simulink library "WECSim_Lib"  (R2019b)
settings: Solver=ode45  StartTime=0.0  StopTime=10.0  RelTol=1e-3  EnableMultiTasking=on
undefined symbols (not defined in the file): body, constraint, mooring, pto, simu, waves, X, Y, Z
libraries: nesl_utility x168, sm_lib x94, vrlib x12
(part 5 of 6)

== system WECSim_Lib/Body Elements/Rigid Body/Hydrodynamic Body/Structure/Motion Sensor ==
  note: Measures the position, velocity, and acceleration of the follower (F) frame relative to the base (B) frame.
      | Ouputs a bus of 3 signals, each signal is a vector length 6.
  Angle : MATLAB Function  TreatAsAtomicUnit=on
  Bus Creator : BusCreator  Inputs=3
  Mux : Mux
  Mux1 : Mux  Inputs=6
  Mux2 : Mux  Inputs=6
  PS-Simulink Converter{,1..15} (16 alike) : nesl_utility/PS-Simulink Converter  PhysicalDomain=network_engine_domain  SubClassName=ps_output  LeftPortType=input  RightPortType=output  PseudoPeriodic=off  Frequencies=[]  Unit=1  AffineConversion=off
  Transform Sensor : sm_lib/Frames and Transforms/Transform Sensor  MeasurementFrame=World  SenseAngle=off  SenseAxis=off  SenseAngle1=off  SenseAngle2=off  SenseAngle3=off  SenseQ=on  SenseR=off  SenseOmegaX=on  SenseOmegaY=on  SenseOmegaZ=on  SenseOmega1=off  SenseOmega2=off  SenseOmega3=off  SenseQDot=off  SenseRDot=off  SenseAlphaX=on  SenseAlphaY=on  SenseAlphaZ=on  SenseAlpha1=off  SenseAlpha2=off  SenseAlpha3=off  SenseQDDot=off  SenseRDDot=off  SenseX=on  SenseY=on  SenseZ=on  SenseRad=off  SenseAzim=off  SenseDist=off  SenseInc=off  SenseXDot=on  SenseYDot=on  SenseZDot=on  SenseRadDot=off  SenseAzimDot=off  SenseDistDot=off  SenseIncDot=off  SenseXDDot=on  SenseYDDot=on  SenseZDDot=on  SenseRadDDot=off  SenseAzimDDot=off  SenseDistDDot=off  SenseIncDDot=off  BlockFunction=simmechanics.library.frames_transforms.transform_sensor
  F : PMIOPort  Side=Right
  B : PMIOPort  Port=2  Side=Left
  Response : Outport
  wires:
  Bus Creator/1 -> Response/1
  PS-Simulink Converter15/1 -> Mux2/3  "az"
  PS-Simulink Converter3/1 -> Mux1/6  "omegaz"
  PS-Simulink Converter11/1 -> Mux1/2  "vy"
  PS-Simulink Converter2/1 -> Mux1/5  "omegay"
  PS-Simulink Converter1/1 -> Mux1/4  "omegax"
  PS-Simulink Converter6/1 -> Mux2/6  "alphaz"
  PS-Simulink Converter5/1 -> Mux2/5  "alphay"
  PS-Simulink Converter9/1 -> Mux/3  "z"
  PS-Simulink Converter8/1 -> Mux/2  "y"
  PS-Simulink Converter7/1 -> Mux/1  "x"
  Angle/1(E) -> Mux/4
  Mux2/1 -> Bus Creator/3  "acc"
  Mux1/1 -> Bus Creator/2  "vel"
  Mux/1 -> Bus Creator/1  "disp"
  PS-Simulink Converter14/1 -> Mux2/2  "ay"
  PS-Simulink Converter13/1 -> Mux2/1  "ax"
  PS-Simulink Converter12/1 -> Mux1/3  "vz"
  PS-Simulink Converter10/1 -> Mux1/1  "vx"
  PS-Simulink Converter4/1 -> Mux2/4  "alphax"
  PS-Simulink Converter/1 -> Angle/1(Q)
  connections:
  PS-Simulink Converter3/LConn1 -- Transform Sensor/RConn5
  PS-Simulink Converter2/LConn1 -- Transform Sensor/RConn4
  PS-Simulink Converter1/LConn1 -- Transform Sensor/RConn3
  PS-Simulink Converter6/LConn1 -- Transform Sensor/RConn8
  PS-Simulink Converter5/LConn1 -- Transform Sensor/RConn7
  PS-Simulink Converter4/LConn1 -- Transform Sensor/RConn6
  PS-Simulink Converter7/LConn1 -- Transform Sensor/RConn9
  PS-Simulink Converter8/LConn1 -- Transform Sensor/RConn10
  PS-Simulink Converter9/LConn1 -- Transform Sensor/RConn11
  PS-Simulink Converter10/LConn1 -- Transform Sensor/RConn12
  PS-Simulink Converter11/LConn1 -- Transform Sensor/RConn13
  PS-Simulink Converter12/LConn1 -- Transform Sensor/RConn14
  PS-Simulink Converter13/LConn1 -- Transform Sensor/RConn15
  PS-Simulink Converter14/LConn1 -- Transform Sensor/RConn16
  PS-Simulink Converter15/LConn1 -- Transform Sensor/RConn17
  Transform Sensor/RConn2 -- PS-Simulink Converter/LConn1
  B/RConn1 -- Transform Sensor/LConn1
  Transform Sensor/RConn1 -- F/RConn1

== system WECSim_Lib/Body Elements/Rigid Body/Hydrodynamic Body/Wave Diffraction and Excitation Force Calculation/Linear Wave Excitation Force Variant Subsystem ==
  note: 1) Add Subsystem or Model blocks as valid variant choices.
      | 2) You cannot connect blocks at this level. At simulation, connectivity is automatically
      | determined, based on the active variant and port name matching.
  In1 : Inport
  Irregular Wave Excitation Force : Subsystem  VariantControl=sv_irregularWaves
  No Wave Excitation Force : Subsystem  VariantControl=sv_noWave
  Regular Wave Excitation Force : Subsystem  VariantControl=sv_regularWaves
  User Defined Wave Excitation Force : Subsystem  VariantControl=sv_udfWaves
  Out1 : Outport

== system WECSim_Lib/Body Elements/Rigid Body/Hydrodynamic Body/Wave Diffraction and Excitation Force Calculation/No Ramp Function ==
  Action Port : ActionPort
  Constant : Constant
  R : Outport  InitialOutput=1
  wires:
  Constant/1 -> R/1

== system WECSim_Lib/Body Elements/Rigid Body/Hydrodynamic Body/Wave Diffraction and Excitation Force Calculation/Nonlinear FK Force Variant Subsystem ==
  note: 1) Add Subsystem or Model blocks as valid variant choices.
      | 2) You cannot connect blocks at this level. At simulation, connectivity is automatically
      | determined, based on the active variant and port name matching.
  In1 : Inport
  In2 : Inport  Port=2
  In3 : Inport  Port=3
  No Nonlinear FroudeKrylov Force : Subsystem  VariantControl=sv_linearHydro
  With Nonlinear FroudeKrylov Force : Subsystem  TreatAsAtomicUnit=on  SystemSampleTime=simu.dtNL  VariantControl=sv_nonlinearHydro
  Out1 : Outport

== system WECSim_Lib/Body Elements/Rigid Body/Hydrodynamic Body/Wave Diffraction and Excitation Force Calculation/Ramp Function ==
  Time : Inport
  Action Port : ActionPort
  Add : Sum
  Add1 : Sum
  Constant : Constant  Value=1/2
  Constant1 : Constant
  Constant2 : Constant  Value=3*pi/2
  Constant3 : Constant  Value=pi
  Divide : Product  Inputs=*/
  Product : Product
  Product1 : Product
  Ramp Time : Constant  Value=simu.rampTime
  Sine Wave Function : Sin  TimeSource=Use external signal  SampleTime=0
  R : Outport
  wires:
  Add/1 -> Product/1
  Sine Wave Function/1 -> Add/2
  Constant1/1 -> Add/1
  Constant/1 -> Product/2
  Product/1 -> R/1
  Time/1 -> Product1/1  "t"
  Ramp Time/1 -> Divide/2  "t_ramp"
  Constant2/1 -> Add1/2  "phase"
  Add1/1 -> Sine Wave Function/1
  Product1/1 -> Add1/1
  Constant3/1 -> Divide/1
  Divide/1 -> Product1/2  "frequency"

== system WECSim_Lib/Body Elements/Rigid Body/Hydrodynamic Body/Wave Radiation Forces Calculation/SS CI and Constant-Damping-CoeVariant Subsystem ==
  note: 1) Add Subsystem or Model blocks as valid variant choices.
      | 2) You cannot connect blocks at this level. At simulation, connectivity is automatically
      | determined, based on the active variant and port name matching.
  In1 : Inport
  In2 : Inport  Port=2
  Constant Coefficients : Subsystem  VariantControl=sv_constantCoeff
  Convolution Integral Calculation : Subsystem  VariantControl=sv_convolution
  "State-Space Calculation " : Subsystem  VariantControl=sv_stateSpace
  Out1 : Outport

== system WECSim_Lib/Body Elements/Rigid Body/Non-Hydro Body/Structure/Motion Sensor ==
  note: Measures the position, velocity, and acceleration of the follower (F) frame relative to the base (B) frame.
      | Ouputs a bus of 3 signals, each signal is a vector length 6.
  Angle : MATLAB Function  TreatAsAtomicUnit=on
  Bus Creator : BusCreator  Inputs=3
  Mux : Mux
  Mux1 : Mux  Inputs=6
  Mux2 : Mux  Inputs=6
  PS-Simulink Converter{,1..15} (16 alike) : nesl_utility/PS-Simulink Converter  PhysicalDomain=network_engine_domain  SubClassName=ps_output  LeftPortType=input  RightPortType=output  PseudoPeriodic=off  Frequencies=[]  Unit=1  AffineConversion=off
  Transform Sensor : sm_lib/Frames and Transforms/Transform Sensor  MeasurementFrame=World  SenseAngle=off  SenseAxis=off  SenseAngle1=off  SenseAngle2=off  SenseAngle3=off  SenseQ=on  SenseR=off  SenseOmegaX=on  SenseOmegaY=on  SenseOmegaZ=on  SenseOmega1=off  SenseOmega2=off  SenseOmega3=off  SenseQDot=off  SenseRDot=off  SenseAlphaX=on  SenseAlphaY=on  SenseAlphaZ=on  SenseAlpha1=off  SenseAlpha2=off  SenseAlpha3=off  SenseQDDot=off  SenseRDDot=off  SenseX=on  SenseY=on  SenseZ=on  SenseRad=off  SenseAzim=off  SenseDist=off  SenseInc=off  SenseXDot=on  SenseYDot=on  SenseZDot=on  SenseRadDot=off  SenseAzimDot=off  SenseDistDot=off  SenseIncDot=off  SenseXDDot=on  SenseYDDot=on  SenseZDDot=on  SenseRadDDot=off  SenseAzimDDot=off  SenseDistDDot=off  SenseIncDDot=off  BlockFunction=simmechanics.library.frames_transforms.transform_sensor
  F : PMIOPort  Side=Right
  B : PMIOPort  Port=2  Side=Left
  Response : Outport
  wires:
  Bus Creator/1 -> Response/1
  PS-Simulink Converter15/1 -> Mux2/3  "az"
  PS-Simulink Converter3/1 -> Mux1/6  "omegaz"
  PS-Simulink Converter11/1 -> Mux1/2  "vy"
  PS-Simulink Converter2/1 -> Mux1/5  "omegay"
  PS-Simulink Converter1/1 -> Mux1/4  "omegax"
  PS-Simulink Converter6/1 -> Mux2/6  "alphaz"
  PS-Simulink Converter5/1 -> Mux2/5  "alphay"
  PS-Simulink Converter9/1 -> Mux/3  "z"
  PS-Simulink Converter8/1 -> Mux/2  "y"
  PS-Simulink Converter7/1 -> Mux/1  "x"
  Angle/1(E) -> Mux/4
  Mux2/1 -> Bus Creator/3  "acc"
  Mux1/1 -> Bus Creator/2  "vel"
  Mux/1 -> Bus Creator/1  "disp"
  PS-Simulink Converter14/1 -> Mux2/2  "ay"
  PS-Simulink Converter13/1 -> Mux2/1  "ax"
  PS-Simulink Converter12/1 -> Mux1/3  "vz"
  PS-Simulink Converter10/1 -> Mux1/1  "vx"
  PS-Simulink Converter4/1 -> Mux2/4  "alphax"
  PS-Simulink Converter/1 -> Angle/1(Q)
  connections:
  PS-Simulink Converter3/LConn1 -- Transform Sensor/RConn5
  PS-Simulink Converter2/LConn1 -- Transform Sensor/RConn4
  PS-Simulink Converter1/LConn1 -- Transform Sensor/RConn3
  PS-Simulink Converter6/LConn1 -- Transform Sensor/RConn8
  PS-Simulink Converter5/LConn1 -- Transform Sensor/RConn7
  PS-Simulink Converter4/LConn1 -- Transform Sensor/RConn6
  PS-Simulink Converter7/LConn1 -- Transform Sensor/RConn9
  PS-Simulink Converter8/LConn1 -- Transform Sensor/RConn10
  PS-Simulink Converter9/LConn1 -- Transform Sensor/RConn11
  PS-Simulink Converter10/LConn1 -- Transform Sensor/RConn12
  PS-Simulink Converter11/LConn1 -- Transform Sensor/RConn13
  PS-Simulink Converter12/LConn1 -- Transform Sensor/RConn14
  PS-Simulink Converter13/LConn1 -- Transform Sensor/RConn15
  PS-Simulink Converter14/LConn1 -- Transform Sensor/RConn16
  PS-Simulink Converter15/LConn1 -- Transform Sensor/RConn17
  Transform Sensor/RConn2 -- PS-Simulink Converter/LConn1
  B/RConn1 -- Transform Sensor/LConn1
  Transform Sensor/RConn1 -- F/RConn1

== system WECSim_Lib/Moorings/MoorDyn/MoorDyn/MoorDyn/Triggered Subsystem ==
  X : Inport
  XD : Inport  Port=2
  Time : Inport  Port=3
  CoupTime : Inport  Port=4
  Trigger : TriggerPort  TriggerType=either  VariantControl=(inherit)
  MATLAB Function : MATLAB Function  TreatAsAtomicUnit=on
  FLines : Outport  PortDimensions=6
  wires:
  CoupTime/1 -> MATLAB Function/4(CoupTime)
  Time/1 -> MATLAB Function/3(Time)
  XD/1 -> MATLAB Function/2(XD)
  MATLAB Function/1(FLines) -> FLines/1
  X/1 -> MATLAB Function/1(X)

== system WECSim_Lib/Body Elements/Rigid Body/Hydrodynamic Body/B2B Subsystem/B2B/CrossCoupling ==
  note: CrossCoupling block is updated by its mask initialization, which is only called on when a simulation is run. 'From' blocks are automatically created and connected based on the number of bodies in the simulation.
  Mux1 : Mux  Inputs=2
  Mux2 : Mux  Inputs=2
  vel : Outport
  acc : Outport  Port=2
  wires:
  [vel1] -> Mux1/1
  Mux1/1 -> vel/1
  [vel2] -> Mux1/2
  [acc1] -> Mux2/1
  Mux2/1 -> acc/1
  [acc2] -> Mux2/2

== system WECSim_Lib/Body Elements/Rigid Body/Hydrodynamic Body/Hydrostatic Restoring Force Calculation/Linear and Nonlinear Restoring Force Variant Subsystem/Linear Hydrostatic Restoring Force  ==
  In1 : Inport
  Add1 : Sum  Inputs=+-
  Add2 : Sum
  Assignment (Add Net Bouyancy Force to Z-Direction) : Assignment  IndexOptions=Index vector (dialog)  Indices=3  OutputSizes=1
  Body Mass : Constant  Value=body.hydroForce.storage.mass
  Constant1 : Constant  Value=[0 0 0 0 0 0]
  Gravity : Constant  Value=simu.g
  Linear Restioring Coefficient Matrix : Constant  Value=body.hydroForce.linearHydroRestCoef
  Product : Product
  Product1 : Product  Inputs=3
  Product2 : Product  Multiplication=Matrix(*)
  Volume : Constant  Value=body.dispVol
  Water Density : Constant  Value=simu.rho
  Out1 : Outport
  wires:
  In1/1 -> Product2/2  "x"
  Body Mass/1 -> Product/2  "m"
  Constant1/1 -> Assignment (Add Net Bouyancy Force to Z-Direction)/1
  Assignment (Add Net Bouyancy Force to Z-Direction)/1 -> Add2/1  "Net Buoyancy Force"
  Add2/1 -> Out1/1  "F_Restoring"
  Volume/1 -> Product1/3  "Vol"
  Gravity/1 -> Product1/2, Product/1  "g"
  Water Density/1 -> Product1/1  "rho"
  Product/1 -> Add1/1  "F_Gravity"
  Product1/1 -> Add1/2  "F_Buoyancy"
  Add1/1 -> Assignment (Add Net Bouyancy Force to Z-Direction)/2
  Product2/1 -> Add2/2  "Linear Restoring Force"
  Linear Restioring Coefficient Matrix/1 -> Product2/1  "K"

== system WECSim_Lib/Body Elements/Rigid Body/Hydrodynamic Body/Hydrostatic Restoring Force Calculation/Linear and Nonlinear Restoring Force Variant Subsystem/Nonlinear Hydrostatic Restoring Force ==
  In1 : Inport
  In2 : Inport  Port=2
  Body Mass2 : Constant  Value=body.hydroForce.storage.mass
  Center of Gravity : Constant  Value=body.cg
  Gravity2 : Constant  Value=simu.g
  Rate Transition : RateTransition
  Rate Transition1 : RateTransition
  Restoring Forces : MATLAB Function  TreatAsAtomicUnit=on  SystemSampleTime=simu.dtNL
  STL areas : Constant  Value=body.bodyGeometry.area
  STL centers : Constant  Value=body.bodyGeometry.center
  STL normal vectors : Constant  Value=body.bodyGeometry.norm
  To Workspace1 : ToWorkspace  VariableName=body1_hspressure_out  SaveFormat=Structure With Time  SampleTime=-1
      settings: Decimation=round(simu.dtOut/simu.dt,0)
  Water Density1 : Constant  Value=simu.rho
  Out1 : Outport
  wires:
  In1/1 -> Restoring Forces/1(x)
  Center of Gravity/1 -> Restoring Forces/8(cg)
  Gravity2/1 -> Restoring Forces/7(g)  "g"
  Water Density1/1 -> Restoring Forces/6(rho)
  STL normal vectors/1 -> Restoring Forces/4(tnorm)
  STL centers/1 -> Restoring Forces/3(center)
  In2/1 -> Restoring Forces/2(elv)
  STL areas/1 -> Restoring Forces/5(area)
  Body Mass2/1 -> Restoring Forces/9(mass)
  Restoring Forces/2(p) -> Rate Transition1/1
  Rate Transition1/1 -> To Workspace1/1
  Restoring Forces/1(f) -> Rate Transition/1
  Rate Transition/1 -> Out1/1

== system WECSim_Lib/Body Elements/Rigid Body/Hydrodynamic Body/Morrison Element and ViscousDampingForceCalculation/Morrison Element Variant Subsystem/Morrison Element Off ==
  Constant : Constant  Value=[0 0 0 0 0 0]
  morison_force : Outport
  wires:
  Constant/1 -> morison_force/1

== system WECSim_Lib/Body Elements/Rigid Body/Hydrodynamic Body/Morrison Element and ViscousDampingForceCalculation/Morrison Element Variant Subsystem/Morrison Element On ==
  note: 1) Add Subsystem or Model blocks as valid variant choices.
      | 2) You cannot connect blocks at this level. At simulation, connectivity is automatically
      | determined, based on the active variant and port name matching.
  displacement : Inport
  velocity : Inport  Port=2
  acceleration : Inport  Port=3
  time : Inport  Port=4
  Irregular Wave Morison Force : Subsystem  TreatAsAtomicUnit=on  SystemSampleTime=simu.dtME  VariantControl=sv_irregularWaves
  No Wave Morison Force : Subsystem  VariantControl=sv_noWave
  Regular Wave Morison Force : Subsystem  TreatAsAtomicUnit=on  SystemSampleTime=simu.dtME  VariantControl=sv_regularWaves
  morison_force : Outport

== system WECSim_Lib/Body Elements/Rigid Body/Hydrodynamic Body/Nonlinear Wave Elevation/Linear or Instantaneous Free Surface/Instantaneous Water Free Surface   ==
  In1 : Inport
  In2 : Inport  Port=2
  Center of Gravity : Constant  Value=body.cg
  Frequency Spacing : Constant  Value=waves.dw
  Instantaneous FS : MATLAB Function  TreatAsAtomicUnit=on
  Ramp Time : Constant  Value=simu.rampTime
  STL Centers : Constant  Value=body.bodyGeometry.center
  Wave Amplitude : Constant  Value=waves.A
  Wave Direction : Constant  Value=waves.waveDir
  Wave Frequency : Constant  Value=waves.w
  Wave Number : Constant  Value=waves.k
  Wave Random Phase : Constant  Value=waves.phase
  Wave Type Number : Constant  Value=waves.typeNum
  Out1 : Outport
  wires:
  Instantaneous FS/1(f) -> Out1/1
  STL Centers/1 -> Instantaneous FS/2(center)
  Center of Gravity/1 -> Instantaneous FS/3(cg)
  Wave Number/1 -> Instantaneous FS/7(k)
  Wave Frequency/1 -> Instantaneous FS/5(w)
  Wave Type Number/1 -> Instantaneous FS/8(typeNum)
  Ramp Time/1 -> Instantaneous FS/10(rampT)
  Wave Random Phase/1 -> Instantaneous FS/11(phaseRand)
  Frequency Spacing/1 -> Instantaneous FS/6(dw)
  In2/1 -> Instantaneous FS/9(t)
  In1/1 -> Instantaneous FS/1(x)
  Wave Direction/1 -> Instantaneous FS/12(waveDir)
  Wave Amplitude/1 -> Instantaneous FS/4(AH)

== system WECSim_Lib/Body Elements/Rigid Body/Hydrodynamic Body/Nonlinear Wave Elevation/Linear or Instantaneous Free Surface/Mean Water Free Surface  ==
  zero : Constant  Value=0
  Out1 : Outport
  wires:
  zero/1 -> Out1/1

== system WECSim_Lib/Body Elements/Rigid Body/Hydrodynamic Body/Wave Diffraction and Excitation Force Calculation/Linear Wave Excitation Force Variant Subsystem/Irregular Wave Excitation Force ==
  note: Calculates the wave force, F_wave, for the case of Irregular Waves.
      |
      | F_wave = sum( F_wave(i))
      |
      | where i = each frequency bin.
  In1 : Inport
  Frequency Spacing Delta Omega : Constant  Value=waves.dw  VectorParams1D=off
  Imaginary Part of Wave Excitation : Constant  Value=body.hydroForce.fExt.im  VectorParams1D=off
  MATLAB Function : MATLAB Function  TreatAsAtomicUnit=on
  Random Phase : Constant  Value=waves.phase  VectorParams1D=off
  Real Part of Wave Excitation : Constant  Value=body.hydroForce.fExt.re  VectorParams1D=off
  Wave Frequency : Constant  Value=waves.w  VectorParams1D=off
  Wave Spectrum : Constant  Value=waves.A  VectorParams1D=off
  Out1 : Outport
  wires:
  Random Phase/1 -> MATLAB Function/5(phaseRand)
  MATLAB Function/1(Fext) -> Out1/1
  Wave Frequency/1 -> MATLAB Function/2(w)
  Imaginary Part of Wave Excitation/1 -> MATLAB Function/4(fExtIM)
  Real Part of Wave Excitation/1 -> MATLAB Function/3(fExtRE)
  Wave Spectrum/1 -> MATLAB Function/1(A)
  In1/1 -> MATLAB Function/7(time)
  Frequency Spacing Delta Omega/1 -> MATLAB Function/6(dw)

== system WECSim_Lib/Body Elements/Rigid Body/Hydrodynamic Body/Wave Diffraction and Excitation Force Calculation/Linear Wave Excitation Force Variant Subsystem/No Wave Excitation Force ==
  Constant : Constant  Value=[0 0 0 0 0 0]
  Out1 : Outport
  wires:
  Constant/1 -> Out1/1

== system WECSim_Lib/Body Elements/Rigid Body/Hydrodynamic Body/Wave Diffraction and Excitation Force Calculation/Linear Wave Excitation Force Variant Subsystem/Regular Wave Excitation Force ==
  note: Calculates the wave force, F_wave, for the case of Regular Waves.
      |
      | F_wave =   A * cos(w * t) * Re{Fext}
      |                -  A * sin(w * t) * Im{Fext}
  In1 : Inport
  Add : Sum
  Add1 : Sum  Inputs=+-
  Constant : Constant  Value=pi/2
  Excitation Imaginary Part : Constant  Value=body.hydroForce.fExt.im(1,:)  VectorParams1D=off
  Excitation Real Part : Constant  Value=body.hydroForce.fExt.re(1,:)  VectorParams1D=off
  Product : Product
  Product1 : Product  Inputs=3
  Product2 : Product  Inputs=3
  Sine Wave Function : Sin  TimeSource=Use external signal  SampleTime=0
  Sine Wave Function1 : Sin  TimeSource=Use external signal  SampleTime=0
  Wave Amplitude : Constant  Value=waves.A(1,:)
  Wave Frequency : Constant  Value=waves.w(1,:)
  Out1 : Outport
  wires:
  In1/1 -> Product/1  "t"
  Wave Frequency/1 -> Product/2  "w"
  Product/1 -> Sine Wave Function/1, Add/1
  Sine Wave Function1/1 -> Product1/3  "cos(w*t)"
  Sine Wave Function/1 -> Product2/2  "sin(wt)"
  Excitation Imaginary Part/1 -> Product2/3  "Im{Fext}"
  Excitation Real Part/1 -> Product1/2  "Re{Fext}"
  Product1/1 -> Add1/1
  Product2/1 -> Add1/2
  Add1/1 -> Out1/1
  Wave Amplitude/1 -> Product2/1, Product1/1  "A"
  Add/1 -> Sine Wave Function1/1
  Constant/1 -> Add/2

== system WECSim_Lib/Body Elements/Rigid Body/Hydrodynamic Body/Wave Diffraction and Excitation Force Calculation/Linear Wave Excitation Force Variant Subsystem/User Defined Wave Excitation Force ==
  note: Calculates the wave force, F_wave, for the case of User Defined Waves.
      |
      | F_wave = convolution calculation [1x6]
  InputWaveForceTimeHistory : FromWorkspace  VariableName=[waves.waveAmpTime(:,1),body.hydroForce.userDefinedFe]  SampleTime=0
  Out1 : Outport
  wires:
  InputWaveForceTimeHistory/1 -> Out1/1

== system WECSim_Lib/Body Elements/Rigid Body/Hydrodynamic Body/Wave Diffraction and Excitation Force Calculation/Nonlinear FK Force Variant Subsystem/No Nonlinear FroudeKrylov Force ==
  Constant : Constant  Value=[0 0 0 0 0 0]
  Out1 : Outport
  wires:
  Constant/1 -> Out1/1

== system WECSim_Lib/Body Elements/Rigid Body/Hydrodynamic Body/Wave Diffraction and Excitation Force Calculation/Nonlinear FK Force Variant Subsystem/With Nonlinear FroudeKrylov Force ==
  In1 : Inport
  In2 : Inport  Port=2
  In3 : Inport  Port=3
  Add : Sum  Inputs=+-
  Center of Gravity : Constant  Value=body.hydroData.properties.cg
  Center of Gravity1 : Constant  Value=body.hydroData.properties.cg
  Constant : Constant  Value=[0 0 0]
  Deep Water Flag : Constant  Value=waves.deepWaterWave
  Diffraction and Excitation Forces : MATLAB Function  TreatAsAtomicUnit=on
  Frequency Spacing : Constant  Value=waves.dw
  Gravity : Constant  Value=simu.g
  Mux : Mux  Inputs=2
  STL Areas : Constant  Value=body.bodyGeometry.area
  STL Centers : Constant  Value=body.bodyGeometry.center
  STL Normal Vectors : Constant  Value=body.bodyGeometry.norm
  To Workspace : ToWorkspace  VariableName=body1_wavenonlinearpressure_out  SaveFormat=Structure With Time  SampleTime=-1
      settings: Decimation=round(simu.dtOut/simu.dt,0)
  To Workspace1 : ToWorkspace  VariableName=body1_wavelinearpressure_out  SaveFormat=Structure With Time  SampleTime=-1
      settings: Decimation=round(simu.dtOut/simu.dt,0)
  Water Density : Constant  Value=simu.rho
  Water Depth : Constant  Value=waves.waterDepth
  Wave Amplitude : Constant  Value=waves.A
  Wave Frequency : Constant  Value=waves.w
  Wave Number : Constant  Value=waves.k
  Wave Random Phase : Constant  Value=waves.phase
  Wave Type Number : Constant  Value=waves.typeNum
  Out1 : Outport
  wires:
  Center of Gravity1/1 -> Diffraction and Excitation Forces/8(cg)
  Diffraction and Excitation Forces/1(f) -> Out1/1
  Gravity/1 -> Diffraction and Excitation Forces/7(g)
  Water Density/1 -> Diffraction and Excitation Forces/6(rho)
  STL Normal Vectors/1 -> Diffraction and Excitation Forces/4(tnorm)
  STL Centers/1 -> Diffraction and Excitation Forces/3(center)
  In3/1 -> Diffraction and Excitation Forces/2(elv)
  In1/1 -> Diffraction and Excitation Forces/16(t)
  Wave Amplitude/1 -> Diffraction and Excitation Forces/9(AH)
  Wave Frequency/1 -> Diffraction and Excitation Forces/10(w)
  Frequency Spacing/1 -> Diffraction and Excitation Forces/11(dw)
  Wave Type Number/1 -> Diffraction and Excitation Forces/15(typeNum)
  Wave Number/1 -> Diffraction and Excitation Forces/14(k)
  Water Depth/1 -> Diffraction and Excitation Forces/12(wDepth)
  Wave Random Phase/1 -> Diffraction and Excitation Forces/17(phaseRand)
  Deep Water Flag/1 -> Diffraction and Excitation Forces/13(deepWaterWave)
  Add/1 -> Diffraction and Excitation Forces/1(x)  "x_cg"
  Mux/1 -> Add/2
  Center of Gravity/1 -> Mux/1  "cg"
  Constant/1 -> Mux/2
  In2/1 -> Add/1
  Diffraction and Excitation Forces/3(wpMeanFS) -> To Workspace1/1
  Diffraction and Excitation Forces/2(wp) -> To Workspace/1
  STL Areas/1 -> Diffraction and Excitation Forces/5(area)

== system WECSim_Lib/Body Elements/Rigid Body/Hydrodynamic Body/Wave Radiation Forces Calculation/SS CI and Constant-Damping-CoeVariant Subsystem/Constant Coefficients ==
  In1 : Inport
  Product : Product  Multiplication=Matrix(*)
  Radiation Damping Matrix : Constant  Value=body.hydroForce.fDamping
  Out1 : Outport
  wires:
  Radiation Damping Matrix/1 -> Product/1
  Product/1 -> Out1/1  "F_Single Frequency"
  In1/1 -> Product/2

== system WECSim_Lib/Body Elements/Rigid Body/Hydrodynamic Body/Wave Radiation Forces Calculation/SS CI and Constant-Damping-CoeVariant Subsystem/Convolution Integral Calculation ==
  In1 : Inport
  MATLAB Function : MATLAB Function  TreatAsAtomicUnit=on  SystemSampleTime=simu.CTTime(2) - simu.CTTime(1)  mask{IRKB=body.hydroForce.irkb, lenJ=length(body.lenJ), CTTime=simu.CTTime}
  Rate Transition : RateTransition
  Reshape : Reshape
  Out1 : Outport
  wires:
  In1/1 -> MATLAB Function/1(v)
  Reshape/1 -> Out1/1
  MATLAB Function/1(F_FM) -> Rate Transition/1
  Rate Transition/1 -> Reshape/1

== system WECSim_Lib/Body Elements/Rigid Body/Hydrodynamic Body/Wave Radiation Forces Calculation/SS CI and Constant-Damping-CoeVariant Subsystem/State-Space Calculation  ==
  In1 : Inport
  State-Space : StateSpace  A=body.hydroForce.ssRadf.A  B=body.hydroForce.ssRadf.B  C=body.hydroForce.ssRadf.C  D=body.hydroForce.ssRadf.D  InitialCondition=0
  Out1 : Outport
  wires:
  In1/1 -> State-Space/1  "x"
  State-Space/1 -> Out1/1

== system WECSim_Lib/Body Elements/Rigid Body/Hydrodynamic Body/Morrison Element and ViscousDampingForceCalculation/Morrison Element Variant Subsystem/Morrison Element On/Irregular Wave Morison Force ==
  displacement : Inport
  velocity : Inport  Port=2
  acceleration : Inport  Port=3
  time : Inport  Port=4
  Area : Constant  Value=body.morrisonElement.characteristicArea  VectorParams1D=off
  Ca : Constant  Value=body.morrisonElement.ca  VectorParams1D=off
  Cd : Constant  Value=body.morrisonElement.cd  VectorParams1D=off
  MESum : Sum  Inputs=+  CollapseMode=Specified dimension
  MorrisonElements : Subsystem  TreatAsAtomicUnit=on
  Reshape : Reshape
  Volume : Constant  Value=body.morrisonElement.VME  VectorParams1D=off
  "r_{g}" : Constant  Value=body.morrisonElement.rgME  VectorParams1D=off
  morison_force : Outport
  wires:
  velocity/1 -> MorrisonElements/2(Vel)
  "r_{g}"/1 -> MorrisonElements/1(r)
  Area/1 -> MorrisonElements/5(A)
  Cd/1 -> MorrisonElements/6(Cd)
  displacement/1 -> MorrisonElements/4(Disp)
  acceleration/1 -> MorrisonElements/3(Accel)
  Volume/1 -> MorrisonElements/7(Vol)
  Ca/1 -> MorrisonElements/8(Ca)
  MorrisonElements/1(Force) -> MESum/1
  Reshape/1 -> morison_force/1
  MESum/1 -> Reshape/1
  time/1 -> MorrisonElements/9(Time)

== system WECSim_Lib/Body Elements/Rigid Body/Hydrodynamic Body/Morrison Element and ViscousDampingForceCalculation/Morrison Element Variant Subsystem/Morrison Element On/No Wave Morison Force ==
  displacement : Inport
  velocity : Inport  Port=2
  acceleration : Inport  Port=3
  time : Inport  Port=4
  Area : Constant  Value=body.morrisonElement.characteristicArea  VectorParams1D=off
  Ca : Constant  Value=body.morrisonElement.ca  VectorParams1D=off
  Cd : Constant  Value=body.morrisonElement.cd  VectorParams1D=off
  MESum : Sum  Inputs=+  CollapseMode=Specified dimension
  MorrisonElements : Subsystem  TreatAsAtomicUnit=on
  Reshape : Reshape
  Volume : Constant  Value=body.morrisonElement.VME  VectorParams1D=off
  "r_{g}" : Constant  Value=body.morrisonElement.rgME  VectorParams1D=off
  morison_force : Outport
  wires:
  "r_{g}"/1 -> MorrisonElements/1(r)
  Area/1 -> MorrisonElements/5(Area)
  Cd/1 -> MorrisonElements/6(Cd)
  MorrisonElements/1(Force) -> MESum/1
  Volume/1 -> MorrisonElements/7(Vol)
  Ca/1 -> MorrisonElements/8(Ca)
  displacement/1 -> MorrisonElements/4(Disp)
  velocity/1 -> MorrisonElements/2(Vel)
  acceleration/1 -> MorrisonElements/3(Accel)
  MESum/1 -> Reshape/1
  Reshape/1 -> morison_force/1
  time/1 -> MorrisonElements/9(Time)

== system WECSim_Lib/Body Elements/Rigid Body/Hydrodynamic Body/Morrison Element and ViscousDampingForceCalculation/Morrison Element Variant Subsystem/Morrison Element On/Regular Wave Morison Force ==
  displacement : Inport
  velocity : Inport  Port=2
  acceleration : Inport  Port=3
  time : Inport  Port=4
  Area : Constant  Value=body.morrisonElement.characteristicArea  VectorParams1D=off
  Ca : Constant  Value=body.morrisonElement.ca  VectorParams1D=off
  Cd : Constant  Value=body.morrisonElement.cd  VectorParams1D=off
  MESum : Sum  Inputs=+  CollapseMode=Specified dimension
  MorrisonElements : Subsystem  TreatAsAtomicUnit=on
  Reshape : Reshape
  Volume : Constant  Value=body.morrisonElement.VME  VectorParams1D=off
  "r_{g}" : Constant  Value=body.morrisonElement.rgME  VectorParams1D=off
  morison_force : Outport
  wires:
  "r_{g}"/1 -> MorrisonElements/1(r)
  Area/1 -> MorrisonElements/5(Area)
  Cd/1 -> MorrisonElements/6(Cd)
  MorrisonElements/1(Force) -> MESum/1
  Volume/1 -> MorrisonElements/7(Vol)
  Ca/1 -> MorrisonElements/8(Ca)
  displacement/1 -> MorrisonElements/4(Disp)
  velocity/1 -> MorrisonElements/2(Vel)
  acceleration/1 -> MorrisonElements/3(Accel)
  MESum/1 -> Reshape/1
  Reshape/1 -> morison_force/1
  time/1 -> MorrisonElements/9(Time)

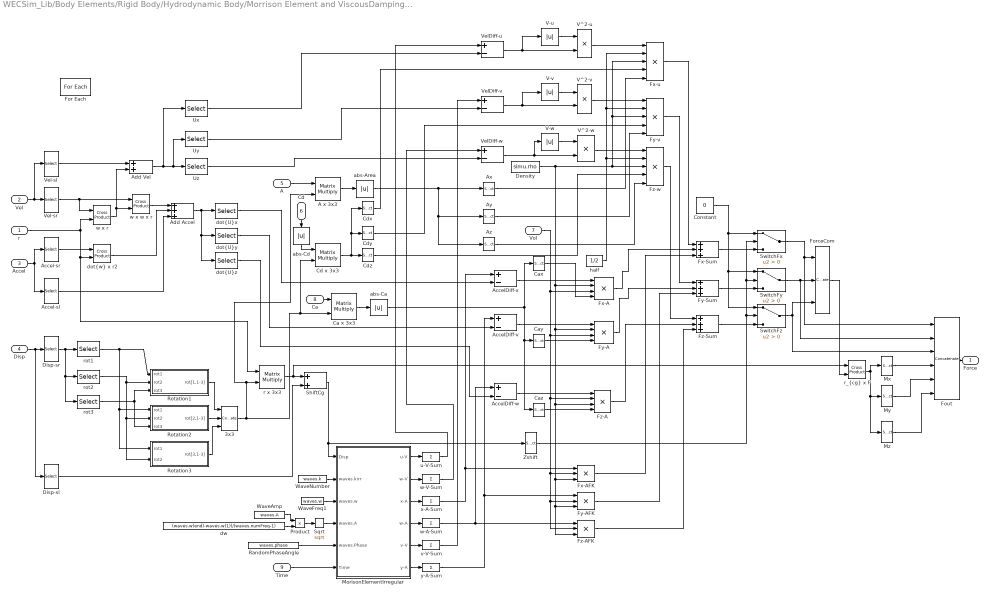
== system WECSim_Lib/Body Elements/Rigid Body/Hydrodynamic Body/Morrison Element and ViscousDampingForceCalculation/Morrison Element Variant Subsystem/Morrison Element On/Irregular Wave Morison Force/MorrisonElements ==
  r : Inport  Partition=on  PartitionDimension=1  PartitionWidth=1  PartitionOffset=0
  Vel : Inport  Port=2
  Accel : Inport  Port=3
  Disp : Inport  Port=4
  A : Inport  Port=5  Partition=on  PartitionDimension=1  PartitionWidth=1  PartitionOffset=0
  Cd : Inport  Port=6  Partition=on  PartitionDimension=1  PartitionWidth=1  PartitionOffset=0
  Vol : Inport  Port=7  Partition=on  PartitionDimension=1  PartitionWidth=1  PartitionOffset=0
  Ca : Inport  Port=8  Partition=on  PartitionDimension=1  PartitionWidth=1  PartitionOffset=0
  Time : Inport  Port=9
  3x3 : Concatenate  NumInputs=3  Mode=Multidimensional array
  A x 3x3 : Product  Multiplication=Matrix(*)
  Accel-sl : Selector  InputPortWidth=6  IndexOptions=Index vector (dialog)  Indices=[1 2 3]  OutputSizes=1
  Accel-sr : Selector  InputPortWidth=6  IndexOptions=Index vector (dialog)  Indices=[4 5 6]  OutputSizes=1
  AccelDiff-v : Sum  Inputs=+-
  AccelDiff-w : Sum  Inputs=+-
  AccelDiff-x : Sum  Inputs=+-
  Add Accel : Sum  Inputs=+++
  Add Vel : Sum
  Ax : Selector  InputPortWidth=3  IndexOptions=Index vector (dialog)  Indices=[1]  OutputSizes=1
  Ay : Selector  InputPortWidth=3  IndexOptions=Index vector (dialog)  Indices=[2]  OutputSizes=1
  Az : Selector  InputPortWidth=3  IndexOptions=Index vector (dialog)  Indices=[3]  OutputSizes=1
  Ca x 3x3 : Product  Multiplication=Matrix(*)
  Cax : Selector  InputPortWidth=3  IndexOptions=Index vector (dialog)  Indices=[1]  OutputSizes=1
  Cay : Selector  InputPortWidth=3  IndexOptions=Index vector (dialog)  Indices=[2]  OutputSizes=1
  Caz : Selector  InputPortWidth=3  IndexOptions=Index vector (dialog)  Indices=[3]  OutputSizes=1
  Cd x 3x3 : Product  Multiplication=Matrix(*)
  Cdx : Selector  InputPortWidth=3  IndexOptions=Index vector (dialog)  Indices=[1]  OutputSizes=1
  Cdy : Selector  InputPortWidth=3  IndexOptions=Index vector (dialog)  Indices=[2]  OutputSizes=1
  Cdz : Selector  InputPortWidth=3  IndexOptions=Index vector (dialog)  Indices=[3]  OutputSizes=1
  Constant : Constant  Value=0
  Density : Constant  Value=simu.rho
  Disp-sl : Selector  InputPortWidth=6  IndexOptions=Index vector (dialog)  Indices=[1 2 3]  OutputSizes=1
  Disp-sr : Selector  InputPortWidth=6  IndexOptions=Index vector (dialog)  Indices=[4 5 6]  OutputSizes=1
  For Each : ForEach  DisableCoverage=on
  ForceCom : Concatenate  NumInputs=3  ConcatenateDimension=2
  Fout : Concatenate  NumInputs=6  Mode=Multidimensional array  ConcatenateDimension=2
  Fx-A : Product  Inputs=4
  Fx-AFK : Product  Inputs=3
  Fx-Sum : Sum  Inputs=+++
  Fx-u : Product  Inputs=5
  Fy-A : Product  Inputs=4
  Fy-AFK : Product  Inputs=3
  Fy-Sum : Sum  Inputs=+++
  Fy-v : Product  Inputs=5
  Fz-A : Product  Inputs=4
  Fz-AFK : Product  Inputs=3
  Fz-Sum : Sum  Inputs=+++
  Fz-w : Product  Inputs=5
  MorisonElementIrregular : Subsystem  TreatAsAtomicUnit=on
  Mx : Selector  InputPortWidth=3  IndexOptions=Index vector (dialog)  Indices=[1]  OutputSizes=1
  My : Selector  InputPortWidth=3  IndexOptions=Index vector (dialog)  Indices=[2]  OutputSizes=1
  Mz : Selector  InputPortWidth=3  IndexOptions=Index vector (dialog)  Indices=[3]  OutputSizes=1
  Product : Product
  RandomPhaseAngle : Constant  Value=waves.phase  VectorParams1D=off
  Rotation1 : Subsystem
  Rotation2 : Subsystem
  Rotation3 : Subsystem
  ShiftCg : Sum
  Sqrt : Sqrt  SaturateOnIntegerOverflow=on
  SwitchFx : Switch  Criteria=u2 > Threshold
  SwitchFy : Switch  Criteria=u2 > Threshold
  SwitchFz : Switch  Criteria=u2 > Threshold
  Ux : Selector  InputPortWidth=3  IndexOptions=Index vector (dialog)  Indices=[1]  OutputSizes=1
  Uy : Selector  InputPortWidth=3  IndexOptions=Index vector (dialog)  Indices=[2]  OutputSizes=1
  Uz : Selector  InputPortWidth=3  IndexOptions=Index vector (dialog)  Indices=[3]  OutputSizes=1
  V-u : Abs
  V-v : Abs
  V-w : Abs
  V^2-u : Product
  V^2-v : Product
  V^2-w : Product
  Vel-sl : Selector  InputPortWidth=6  IndexOptions=Index vector (dialog)  Indices=[1 2 3]  OutputSizes=1
  "Vel-sr " : Selector  InputPortWidth=6  IndexOptions=Index vector (dialog)  Indices=[4 5 6]  OutputSizes=1
  VelDiff-u : Sum  Inputs=+-
  VelDiff-v : Sum  Inputs=+-
  VelDiff-w : Sum  Inputs=+-
  WaveAmp : Constant  Value=waves.A  VectorParams1D=off
  WaveFreq1 : Constant  Value=waves.w  VectorParams1D=off
  WaveNumber : Constant  Value=waves.k  VectorParams1D=off
  Zshift : Selector  InputPortWidth=3  IndexOptions=Index vector (dialog)  Indices=[3]  OutputSizes=1
  abs-Area : Abs
  abs-Ca : Abs
  abs-Cd : Abs
  "dot{U}x" : Selector  InputPortWidth=3  IndexOptions=Index vector (dialog)  Indices=[1]  OutputSizes=1
  "dot{U}y" : Selector  InputPortWidth=3  IndexOptions=Index vector (dialog)  Indices=[2]  OutputSizes=1
  "dot{U}z" : Selector  InputPortWidth=3  IndexOptions=Index vector (dialog)  Indices=[3]  OutputSizes=1
  "dot{w} x r2" : vrlib/Utilities/Cross Product
      settings: SourceProductName=Simulink
  dw : Constant  Value=(waves.w(end)-waves.w(1))/(waves.numFreq-1)  VectorParams1D=off
  half : Constant  Value=1/2
  r x 3x3 : Product  Multiplication=Matrix(*)
  "r_{cg} x F" : vrlib/Utilities/Cross Product
      settings: SourceProductName=Simulink
  rot1 : Selector  InputPortWidth=3  IndexOptions=Index vector (dialog)  Indices=[1]  OutputSizes=1
  rot2 : Selector  InputPortWidth=3  IndexOptions=Index vector (dialog)  Indices=[2]  OutputSizes=1
  rot3 : Selector  InputPortWidth=3  IndexOptions=Index vector (dialog)  Indices=[3]  OutputSizes=1
  u-V-Sum : Sum  Inputs=+  CollapseMode=Specified dimension
  v-V-Sum : Sum  Inputs=+  CollapseMode=Specified dimension
  w x r : vrlib/Utilities/Cross Product
      settings: SourceProductName=Simulink
  w x w x r : vrlib/Utilities/Cross Product
      settings: SourceProductName=Simulink
  w-A-Sum : Sum  Inputs=+  CollapseMode=Specified dimension
  w-V-Sum : Sum  Inputs=+  CollapseMode=Specified dimension
  x-A-Sum : Sum  Inputs=+  CollapseMode=Specified dimension
  y-A-Sum : Sum  Inputs=+  CollapseMode=Specified dimension
  Force : Outport  PortDimensions=[1 6]  ConcatenationDimension=1
  wires:
  Vel/1 -> Vel-sl/1, "Vel-sr "/1
  w x r/1 -> Add Vel/2, w x w x r/2
  w x w x r/1 -> Add Accel/1
  "Vel-sr "/1 -> w x w x r/1, w x r/1
  r/1 -> r x 3x3/1, "dot{w} x r2"/2, w x r/2
  Accel/1 -> Accel-sl/1, Accel-sr/1
  Accel-sr/1 -> "dot{w} x r2"/1
  "dot{w} x r2"/1 -> Add Accel/2
  Accel-sl/1 -> Add Accel/3
  Add Accel/1 -> "dot{U}z"/1, "dot{U}y"/1, "dot{U}x"/1
  Vel-sl/1 -> Add Vel/1
  Disp/1 -> Disp-sl/1, Disp-sr/1
  Disp-sr/1 -> rot3/1, rot2/1, rot1/1
  rot3/1 -> Rotation2/3(rot3), Rotation1/3(rot3)
  rot1/1 -> Rotation3/1(rot1), Rotation2/1(rot1), Rotation1/1(rot1)
  rot2/1 -> Rotation3/2(rot2), Rotation2/2(rot2), Rotation1/2(rot2)
  Rotation2/1(rot[2,1-3]) -> 3x3/2
  Rotation1/1(rot[1,1-3]) -> 3x3/1
  Rotation3/1(rot[3,1-3]) -> 3x3/3
  r x 3x3/1 -> "r_{cg} x F"/1, ShiftCg/1
  Disp-sl/1 -> ShiftCg/2
  ShiftCg/1 -> MorisonElementIrregular/1(Disp), Zshift/1
  "dot{U}y"/1 -> AccelDiff-v/2
  "dot{U}x"/1 -> AccelDiff-x/2
  x-A-Sum/1 -> Fx-AFK/1, AccelDiff-x/1
  "dot{U}z"/1 -> AccelDiff-w/2
  Add Vel/1 -> Ux/1, Uy/1, Uz/1
  Uy/1 -> VelDiff-v/2
  Ux/1 -> VelDiff-u/2
  Uz/1 -> VelDiff-w/2
  u-V-Sum/1 -> VelDiff-u/1
  w-V-Sum/1 -> VelDiff-w/1
  VelDiff-w/1 -> V^2-w/2, V-w/1
  V^2-u/1 -> Fx-u/1
  half/1 -> Fz-w/2, Fy-v/2, Fx-u/2
  Density/1 -> Fy-A/2, Fy-AFK/3, Fz-AFK/3, Fx-AFK/3, Fz-A/3, Fx-A/2, Fy-v/3, Fx-u/3, Fz-w/3
  V^2-w/1 -> Fz-w/1
  AccelDiff-x/1 -> Fx-A/1
  Vol/1 -> Fy-A/3, Fy-AFK/2, Fz-AFK/2, Fx-AFK/2, Fz-A/2, Fx-A/3
  AccelDiff-w/1 -> Fz-A/1
  w-A-Sum/1 -> AccelDiff-w/1, Fz-AFK/1
  Fx-u/1 -> Fx-Sum/1
  Fx-A/1 -> Fx-Sum/2
  Fx-AFK/1 -> Fx-Sum/3
  Fz-w/1 -> Fz-Sum/1
  Fz-A/1 -> Fz-Sum/2
  Fz-AFK/1 -> Fz-Sum/3
  Constant/1 -> SwitchFy/1, SwitchFz/1, SwitchFx/1
  "r_{cg} x F"/1 -> Mz/1, My/1, Mx/1
  Mx/1 -> Fout/4
  My/1 -> Fout/5
  Mz/1 -> Fout/6
  3x3/1 -> A x 3x3/2, r x 3x3/2, Ca x 3x3/2, Cd x 3x3/2
  VelDiff-u/1 -> V-u/1, V^2-u/2
  Zshift/1 -> SwitchFy/2, SwitchFx/2, SwitchFz/2
  SwitchFz/1 -> ForceCom/3, Fout/3
  SwitchFx/1 -> Fout/1, ForceCom/1
  Fx-Sum/1 -> SwitchFx/3
  Fz-Sum/1 -> SwitchFz/3
  Az/1 -> Fz-w/5
  A/1 -> A x 3x3/1
  Ax/1 -> Fx-u/5
  Cdx/1 -> Fx-u/4
  Cdz/1 -> Fz-w/4
  A x 3x3/1 -> abs-Area/1
  abs-Area/1 -> Ay/1, Az/1, Ax/1
  ForceCom/1 -> "r_{cg} x F"/2
  Fout/1 -> Force/1
  Caz/1 -> Fz-A/4
  Cax/1 -> Fx-A/4
  Cd/1 -> abs-Cd/1
  Cd x 3x3/1 -> Cdz/1, Cdy/1, Cdx/1
  Ca/1 -> Ca x 3x3/1
  Ca x 3x3/1 -> abs-Ca/1
  WaveNumber/1 -> MorisonElementIrregular/2(waves.kirr)
  WaveFreq1/1 -> MorisonElementIrregular/3(waves.w)
  RandomPhaseAngle/1 -> MorisonElementIrregular/5(waves.Phase)
  MorisonElementIrregular/1(u-V) -> u-V-Sum/1
  WaveAmp/1 -> Product/1
  dw/1 -> Product/2
  Product/1 -> Sqrt/1
  Sqrt/1 -> MorisonElementIrregular/4(waves.A)
  MorisonElementIrregular/2(w-V) -> w-V-Sum/1
  MorisonElementIrregular/3(x-A) -> x-A-Sum/1
  MorisonElementIrregular/4(w-A) -> w-A-Sum/1
  V-u/1 -> V^2-u/1
  MorisonElementIrregular/5(v-V) -> v-V-Sum/1
  MorisonElementIrregular/6(y-A) -> y-A-Sum/1
  V-w/1 -> V^2-w/1
  VelDiff-v/1 -> V-v/1, V^2-v/2
  V-v/1 -> V^2-v/1
  v-V-Sum/1 -> VelDiff-v/1
  V^2-v/1 -> Fy-v/1
  Ay/1 -> Fy-v/5
  Cdy/1 -> Fy-v/4
  SwitchFy/1 -> Fout/2, ForceCom/2
  Fy-Sum/1 -> SwitchFy/3
  Fy-v/1 -> Fy-Sum/1
  y-A-Sum/1 -> Fy-AFK/1, AccelDiff-v/1
  Cay/1 -> Fy-A/4
  AccelDiff-v/1 -> Fy-A/1
  Fy-A/1 -> Fy-Sum/2
  Fy-AFK/1 -> Fy-Sum/3
  abs-Ca/1 -> Cax/1, Caz/1, Cay/1
  abs-Cd/1 -> Cd x 3x3/1
  Time/1 -> MorisonElementIrregular/6(Time)

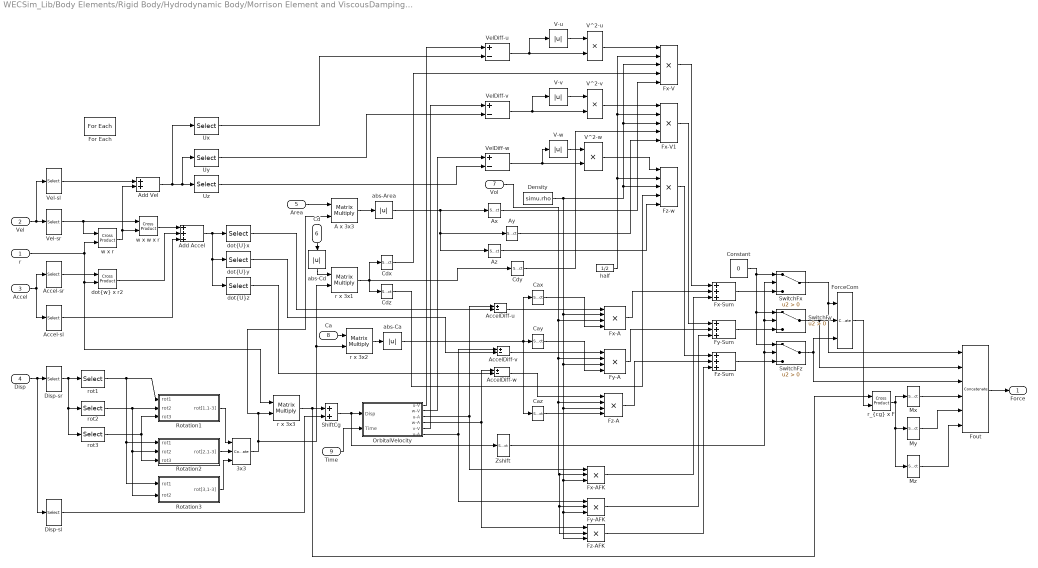
== system WECSim_Lib/Body Elements/Rigid Body/Hydrodynamic Body/Morrison Element and ViscousDampingForceCalculation/Morrison Element Variant Subsystem/Morrison Element On/No Wave Morison Force/MorrisonElements ==
  r : Inport  Partition=on  PartitionDimension=1  PartitionWidth=1  PartitionOffset=0
  Vel : Inport  Port=2
  Accel : Inport  Port=3
  Disp : Inport  Port=4
  Area : Inport  Port=5  Partition=on  PartitionDimension=1  PartitionWidth=1  PartitionOffset=0
  Cd : Inport  Port=6  Partition=on  PartitionDimension=1  PartitionWidth=1  PartitionOffset=0
  Vol : Inport  Port=7  Partition=on  PartitionDimension=1  PartitionWidth=1  PartitionOffset=0
  Ca : Inport  Port=8  Partition=on  PartitionDimension=1  PartitionWidth=1  PartitionOffset=0
  Time : Inport  Port=9
  3x3 : Concatenate  NumInputs=3  Mode=Multidimensional array
  A x 3x3 : Product  Multiplication=Matrix(*)
  Accel-sl : Selector  InputPortWidth=6  IndexOptions=Index vector (dialog)  Indices=[1 2 3]  OutputSizes=1
  Accel-sr : Selector  InputPortWidth=6  IndexOptions=Index vector (dialog)  Indices=[4 5 6]  OutputSizes=1
  AccelDiff-u : Sum  Inputs=+-
  AccelDiff-v : Sum  Inputs=+-
  AccelDiff-w : Sum  Inputs=+-
  Add Accel : Sum  Inputs=+++
  Add Vel : Sum
  Ax : Selector  InputPortWidth=3  IndexOptions=Index vector (dialog)  Indices=[1]  OutputSizes=1
  Ay : Selector  InputPortWidth=3  IndexOptions=Index vector (dialog)  Indices=[2]  OutputSizes=1
  Az : Selector  InputPortWidth=3  IndexOptions=Index vector (dialog)  Indices=[3]  OutputSizes=1
  Cax : Selector  InputPortWidth=3  IndexOptions=Index vector (dialog)  Indices=[1]  OutputSizes=1
  Cay : Selector  InputPortWidth=3  IndexOptions=Index vector (dialog)  Indices=[2]  OutputSizes=1
  Caz : Selector  InputPortWidth=3  IndexOptions=Index vector (dialog)  Indices=[3]  OutputSizes=1
  Cdx : Selector  InputPortWidth=3  IndexOptions=Index vector (dialog)  Indices=[1]  OutputSizes=1
  Cdy : Selector  InputPortWidth=3  IndexOptions=Index vector (dialog)  Indices=[2]  OutputSizes=1
  Cdz : Selector  InputPortWidth=3  IndexOptions=Index vector (dialog)  Indices=[3]  OutputSizes=1
  Constant : Constant  Value=0
  Density : Constant  Value=simu.rho
  Disp-sl : Selector  InputPortWidth=6  IndexOptions=Index vector (dialog)  Indices=[1 2 3]  OutputSizes=1
  Disp-sr : Selector  InputPortWidth=6  IndexOptions=Index vector (dialog)  Indices=[4 5 6]  OutputSizes=1
  For Each : ForEach  DisableCoverage=on
  ForceCom : Concatenate  NumInputs=3  ConcatenateDimension=2
  Fout : Concatenate  NumInputs=6  Mode=Multidimensional array  ConcatenateDimension=2
  Fx-A : Product  Inputs=4
  Fx-AFK : Product  Inputs=3
  Fx-Sum : Sum  Inputs=+++
  Fx-V : Product  Inputs=5
  Fx-V1 : Product  Inputs=5
  Fy-A : Product  Inputs=4
  Fy-AFK : Product  Inputs=3
  Fy-Sum : Sum  Inputs=+++
  Fz-A : Product  Inputs=4
  Fz-AFK : Product  Inputs=3
  Fz-Sum : Sum  Inputs=+++
  Fz-w : Product  Inputs=5
  Mx : Selector  InputPortWidth=3  IndexOptions=Index vector (dialog)  Indices=[1]  OutputSizes=1
  My : Selector  InputPortWidth=3  IndexOptions=Index vector (dialog)  Indices=[2]  OutputSizes=1
  Mz : Selector  InputPortWidth=3  IndexOptions=Index vector (dialog)  Indices=[3]  OutputSizes=1
  OrbitalVelocity : Subsystem
  Rotation1 : Subsystem
  Rotation2 : Subsystem
  Rotation3 : Subsystem
  ShiftCg : Sum
  SwitchFx : Switch  Criteria=u2 > Threshold
  SwitchFy : Switch  Criteria=u2 > Threshold
  SwitchFz : Switch  Criteria=u2 > Threshold
  Ux : Selector  InputPortWidth=3  IndexOptions=Index vector (dialog)  Indices=[1]  OutputSizes=1
  Uy : Selector  InputPortWidth=3  IndexOptions=Index vector (dialog)  Indices=[2]  OutputSizes=1
  Uz : Selector  InputPortWidth=3  IndexOptions=Index vector (dialog)  Indices=[3]  OutputSizes=1
  V-u : Abs
  V-v : Abs
  V-w : Abs
  V^2-u : Product
  V^2-v : Product
  V^2-w : Product
  Vel-sl : Selector  InputPortWidth=6  IndexOptions=Index vector (dialog)  Indices=[1 2 3]  OutputSizes=1
  "Vel-sr " : Selector  InputPortWidth=6  IndexOptions=Index vector (dialog)  Indices=[4 5 6]  OutputSizes=1
  VelDiff-u : Sum  Inputs=+-
  VelDiff-v : Sum  Inputs=+-
  VelDiff-w : Sum  Inputs=+-
  Zshift : Selector  InputPortWidth=3  IndexOptions=Index vector (dialog)  Indices=[3]  OutputSizes=1
  abs-Area : Abs
  abs-Ca : Abs
  abs-Cd : Abs
  "dot{U}x" : Selector  InputPortWidth=3  IndexOptions=Index vector (dialog)  Indices=[1]  OutputSizes=1
  "dot{U}y" : Selector  InputPortWidth=3  IndexOptions=Index vector (dialog)  Indices=[2]  OutputSizes=1
  "dot{U}z" : Selector  InputPortWidth=3  IndexOptions=Index vector (dialog)  Indices=[3]  OutputSizes=1
  "dot{w} x r2" : vrlib/Utilities/Cross Product
      settings: SourceProductName=Simulink
  half : Constant  Value=1/2
  r x 3x1 : Product  Multiplication=Matrix(*)
  r x 3x2 : Product  Multiplication=Matrix(*)
  r x 3x3 : Product  Multiplication=Matrix(*)
  "r_{cg} x F" : vrlib/Utilities/Cross Product
      settings: SourceProductName=Simulink
  rot1 : Selector  InputPortWidth=3  IndexOptions=Index vector (dialog)  Indices=[1]  OutputSizes=1
  rot2 : Selector  InputPortWidth=3  IndexOptions=Index vector (dialog)  Indices=[2]  OutputSizes=1
  rot3 : Selector  InputPortWidth=3  IndexOptions=Index vector (dialog)  Indices=[3]  OutputSizes=1
  w x r : vrlib/Utilities/Cross Product
      settings: SourceProductName=Simulink
  w x w x r : vrlib/Utilities/Cross Product
      settings: SourceProductName=Simulink
  Force : Outport  PortDimensions=[1 6]  ConcatenationDimension=1
  wires:
  Vel/1 -> Vel-sl/1, "Vel-sr "/1
  w x r/1 -> Add Vel/2, w x w x r/2
  w x w x r/1 -> Add Accel/1
  "Vel-sr "/1 -> w x w x r/1, w x r/1
  r/1 -> r x 3x3/1, "dot{w} x r2"/2, w x r/2
  Accel/1 -> Accel-sl/1, Accel-sr/1
  Accel-sr/1 -> "dot{w} x r2"/1
  "dot{w} x r2"/1 -> Add Accel/2
  Accel-sl/1 -> Add Accel/3
  Add Accel/1 -> "dot{U}z"/1, "dot{U}y"/1, "dot{U}x"/1
  Vel-sl/1 -> Add Vel/1
  Disp/1 -> Disp-sl/1, Disp-sr/1
  Disp-sr/1 -> rot3/1, rot2/1, rot1/1
  rot3/1 -> Rotation2/3(rot3), Rotation1/3(rot3)
  rot1/1 -> Rotation3/1(rot1), Rotation2/1(rot1), Rotation1/1(rot1)
  rot2/1 -> Rotation3/2(rot2), Rotation2/2(rot2), Rotation1/2(rot2)
  Rotation2/1(rot[2,1-3]) -> 3x3/2
  Rotation1/1(rot[1,1-3]) -> 3x3/1
  Rotation3/1(rot[3,1-3]) -> 3x3/3
  r x 3x3/1 -> "r_{cg} x F"/1, ShiftCg/1
  Disp-sl/1 -> ShiftCg/2
  ShiftCg/1 -> Zshift/1, OrbitalVelocity/1(Disp)
  "dot{U}y"/1 -> AccelDiff-v/2
  "dot{U}x"/1 -> AccelDiff-u/2
  OrbitalVelocity/3(u-A) -> AccelDiff-u/1, Fx-AFK/1
  "dot{U}z"/1 -> AccelDiff-w/2
  Add Vel/1 -> Uy/1, Uz/1, Ux/1
  Uy/1 -> VelDiff-v/2
  Ux/1 -> VelDiff-u/2
  Uz/1 -> VelDiff-w/2
  OrbitalVelocity/1(u-V) -> VelDiff-u/1
  OrbitalVelocity/2(w-V) -> VelDiff-w/1
  VelDiff-w/1 -> V-w/1, V^2-w/2
  V^2-u/1 -> Fx-V/1
  half/1 -> Fz-w/2, Fx-V1/2, Fx-V/2
  Density/1 -> Fy-A/3, Fy-AFK/3, Fz-AFK/3, Fx-AFK/3, Fz-A/3, Fx-A/2, Fz-w/3, Fx-V1/3, Fx-V/3
  V^2-w/1 -> Fz-w/1
  AccelDiff-u/1 -> Fx-A/1
  Vol/1 -> Fy-A/2, Fy-AFK/2, Fz-AFK/2, Fx-AFK/2, Fz-A/2, Fx-A/3
  AccelDiff-w/1 -> Fz-A/1
  OrbitalVelocity/4(w-A) -> Fz-AFK/1, AccelDiff-w/1
  Fx-V/1 -> Fx-Sum/1
  Fx-A/1 -> Fx-Sum/2
  Fx-AFK/1 -> Fx-Sum/3
  Fz-w/1 -> Fz-Sum/1
  Fz-A/1 -> Fz-Sum/2
  Fz-AFK/1 -> Fz-Sum/3
  "r_{cg} x F"/1 -> Mz/1, My/1, Mx/1
  Mx/1 -> Fout/4
  My/1 -> Fout/5
  Mz/1 -> Fout/6
  3x3/1 -> A x 3x3/2, r x 3x3/2, r x 3x2/2, r x 3x1/2
  V-u/1 -> V^2-u/1
  VelDiff-u/1 -> V-u/1, V^2-u/2
  Zshift/1 -> SwitchFy/2, SwitchFx/2, SwitchFz/2
  SwitchFz/1 -> ForceCom/3, Fout/3
  SwitchFx/1 -> Fout/1, ForceCom/1
  Fx-Sum/1 -> SwitchFx/3
  Fz-Sum/1 -> SwitchFz/3
  Az/1 -> Fz-w/5
  Area/1 -> A x 3x3/1
  Ax/1 -> Fx-V/5
  Cdx/1 -> Fx-V/4
  Cdz/1 -> Fz-w/4
  A x 3x3/1 -> abs-Area/1
  abs-Area/1 -> Ay/1, Az/1, Ax/1
  ForceCom/1 -> "r_{cg} x F"/2
  Fout/1 -> Force/1
  Caz/1 -> Fz-A/4
  Cax/1 -> Fx-A/4
  Cd/1 -> abs-Cd/1
  r x 3x1/1 -> Cdy/1, Cdz/1, Cdx/1
  Ca/1 -> r x 3x2/1
  r x 3x2/1 -> abs-Ca/1
  OrbitalVelocity/6(v-A) -> AccelDiff-v/1, Fy-AFK/1
  V^2-v/1 -> Fx-V1/1
  V-v/1 -> V^2-v/1
  VelDiff-v/1 -> V-v/1, V^2-v/2
  OrbitalVelocity/5(v-V) -> VelDiff-v/1
  Ay/1 -> Fx-V1/5
  Cdy/1 -> Fx-V1/4
  SwitchFy/1 -> Fout/2, ForceCom/2
  Fy-Sum/1 -> SwitchFy/3
  Fy-AFK/1 -> Fy-Sum/3
  AccelDiff-v/1 -> Fy-A/1
  Cay/1 -> Fy-A/4
  Fy-A/1 -> Fy-Sum/2
  Fx-V1/1 -> Fy-Sum/1
  Constant/1 -> SwitchFy/1, SwitchFz/1, SwitchFx/1
  V-w/1 -> V^2-w/1
  abs-Ca/1 -> Cax/1, Cay/1, Caz/1
  abs-Cd/1 -> r x 3x1/1
  Time/1 -> OrbitalVelocity/2(Time)
